simulink model "SF5_2_4_jc0531_2_C"  (R2016b)
settings: Solver=VariableStepAuto  StartTime=0.0  StopTime=inf  RelTol=1e-3  EnableMultiTasking=on
settings Model: Creator=amyyang  LastModifiedBy=amyyang
settings DataIOCC: LimitDataPoints=on
settings OptimizationCC: LifeSpan=inf
settings DebuggingCC: AllowSymbolicDim=off  SFUnexpectedBacktrackingDiag=warning  SFNoUnconditionalDefaultTransitionDiag=warning  SFExecutionAtInitializationDiag=none
settings ModelReferenceCC: PropagateSignalLabelsOutOfModel=off
settings GRTTargetCC: TargetLangStandard=C89/C90 (ANSI)
settings ConfigComp: CovMetricSettings=dw  CovHtmlReporting=on  CovSaveCumulativeToWorkspaceVar=on  CovSaveSingleToWorkspaceVar=on  CovExternalEMLEnable=off

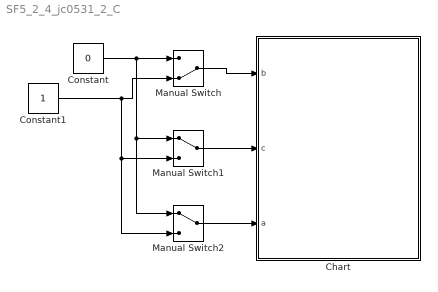
== system SF5_2_4_jc0531_2_C ==
  Chart : Stateflow chart  TreatAsAtomicUnit=on
  Constant : Constant  Value=0
  Constant1 : Constant
  Manual Switch : ManualSwitch  CurrentSetting=0
  Manual Switch1 : ManualSwitch
  Manual Switch2 : ManualSwitch
  wires:
  Manual Switch/1 -> Chart/1(b)
  Constant1/1 -> Manual Switch2/2, Manual Switch1/2, Manual Switch/2
  Constant/1 -> Manual Switch2/1, Manual Switch1/1, Manual Switch/1
  Manual Switch1/1 -> Chart/2(c)
  Manual Switch2/1 -> Chart/3(a)

== stateflow chart SF5_2_4_jc0531_2_C/Chart ==
  state B
    state BB1
    state BB2
    (default) -> (junction 14)
    (junction 14) -> BB1 [order 1] : [ a>0]
    (junction 14) -> (junction 15) [order 2]
    BB1 -> BB2 : after(5,sec)
    BB2 -> BB1 : after(5,sec)
    (junction 15) -> BB2 : [ c>0]
  state A
  (default) -> A
  A -> B : [ b > 0]
  data: b input; c input; a input
